simulink model "second_order_demo"  (R2017a)
settings: Solver=VariableStepAuto  StartTime=0.0  StopTime=500  RelTol=1e-3
settings Model: Creator=DELL  LastModifiedBy=DELL
settings DataIOCC: SaveState=on  InspectSignalLogs=on  LoggingToFile=on

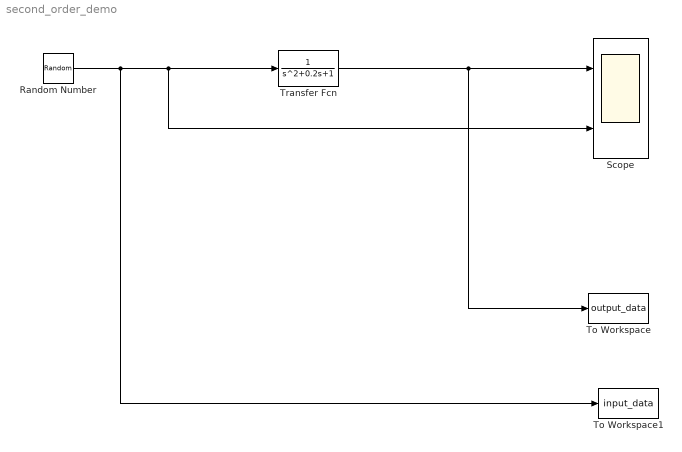
== system second_order_demo ==
  Random Number : RandomNumber  SampleTime=0.001
  Scope : Scope  NumInputPorts=2
  To Workspace : ToWorkspace  VariableName=output_data  SaveFormat=Timeseries  SampleTime=-1
  To Workspace1 : ToWorkspace  VariableName=input_data  SaveFormat=Timeseries  SampleTime=-1
  Transfer Fcn : TransferFcn  Denominator=[1 0.2 1]
  wires:
  Random Number/1 -> To Workspace1/1, Scope/2, Transfer Fcn/1
  Transfer Fcn/1 -> To Workspace/1, Scope/1
